simulink model "OttoCycle"  (R2018a)
settings: Solver=VariableStepAuto  StartTime=0.0  StopTime=0  RelTol=1e-3
settings Model: Creator=josefl  LastModifiedBy=josefl

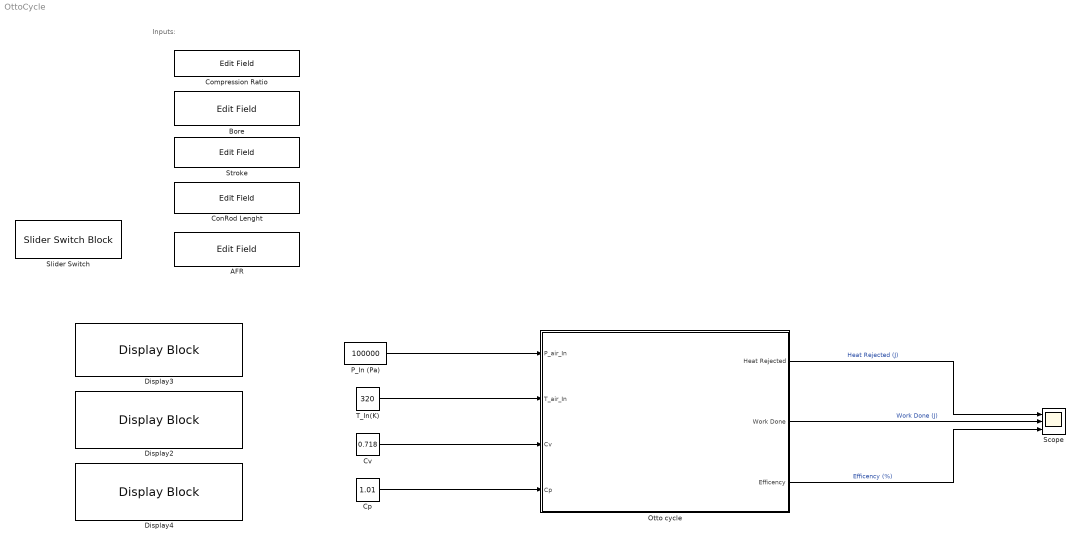
== system OttoCycle ==
  note: Inputs:
  AFR : EditField  WebBlockId=118  LabelPosition=Hide  Alignment=Center
  Bore : EditField  WebBlockId=61  LabelPosition=Hide  Alignment=Center
  "Compression Ratio " : EditField  WebBlockId=60  LabelPosition=Hide  Alignment=Center
  ConRod Lenght : EditField  WebBlockId=93  LabelPosition=Hide  Alignment=Center
  "Cp " : Constant  Value=1.01
  Cv : Constant  Value=0.718
  Display2 : DisplayBlock  WebBlockId=86
  Display3 : DisplayBlock  WebBlockId=87
  Display4 : DisplayBlock  WebBlockId=88
  "Otto cycle " : Subsystem
  "P_In (Pa) " : Constant  Value=100000
  Scope : Scope  NumInputPorts=3
  Slider Switch : SliderSwitchBlock  WebBlockId=121
      settings: Values={{'Off', 'On'}, [0.8 2]}
  "Stroke " : EditField  WebBlockId=62  LabelPosition=Hide  Alignment=Center
  "T_In(K) " : Constant  Value=320
  wires:
  Cv/1 -> "Otto cycle "/3(Cv)
  "Cp "/1 -> "Otto cycle "/4("Cp ")
  "Otto cycle "/1("Heat Rejected ") -> Scope/1  "Heat Rejected (J)"
  "Otto cycle "/2(Work Done) -> Scope/2  "Work Done (J)"
  "Otto cycle "/3(Efficency) -> Scope/3  "Efficency (%)"
  "T_In(K) "/1 -> "Otto cycle "/2("T_air_In ")
  "P_In (Pa) "/1 -> "Otto cycle "/1("P_air_In ")

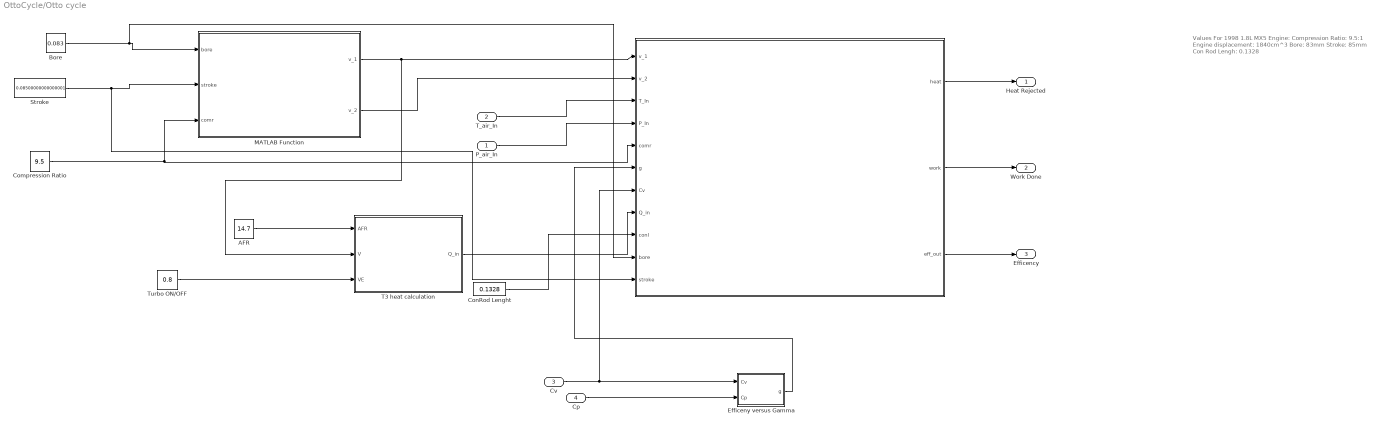
== system OttoCycle/Otto cycle  ==
  note: Values For 1998 1.8L MX5 Engine:
      | Compression Ratio: 9.5:1
      | Engine displacement: 1840cm^3
      | Bore: 83mm
      | Stroke: 85mm
      | Con Rod Lengh: 0.1328
  "P_air_In " : Inport
  "T_air_In " : Inport  Port=2
  Cv : Inport  Port=3
  "Cp " : Inport  Port=4
  " " : MATLAB Function  TreatAsAtomicUnit=on
  AFR : Constant  Value=14.7  VectorParams1D=off
  "Bore " : Constant  Value=0.083
  "Compression Ratio " : Constant  Value=9.5
  ConRod Lenght : Constant  Value=0.1328
  "Efficeny versus Gamma " : MATLAB Function  TreatAsAtomicUnit=on
  MATLAB Function : MATLAB Function  TreatAsAtomicUnit=on
  "Stroke " : Constant  Value=0.08500000000000001
  "T3 heat calculation " : MATLAB Function  TreatAsAtomicUnit=on
  "Turbo ON/OFF " : Constant  Value=0.8
  "Heat Rejected " : Outport
  Work Done : Outport  Port=2
  Efficency : Outport  Port=3
  wires:
  "Compression Ratio "/1 -> " "/5(comr), MATLAB Function/3(comr)
  "P_air_In "/1 -> " "/4(P_In)
  "T_air_In "/1 -> " "/3(T_In)
  Cv/1 -> " "/7(Cv), "Efficeny versus Gamma "/1(Cv)
  ConRod Lenght/1 -> " "/9(conl)
  "Cp "/1 -> "Efficeny versus Gamma "/2(Cp)
  " "/1(heat) -> "Heat Rejected "/1
  " "/2(work) -> Work Done/1
  " "/3(eff_out) -> Efficency/1
  "Efficeny versus Gamma "/1(g) -> " "/6(g)
  "T3 heat calculation "/1(Q_in) -> " "/8(Q_in)
  AFR/1 -> "T3 heat calculation "/1(AFR)
  "Turbo ON/OFF "/1 -> "T3 heat calculation "/3(VE)
  "Stroke "/1 -> " "/11(stroke), MATLAB Function/2(stroke)
  "Bore "/1 -> " "/10(bore), MATLAB Function/1(bore)
  MATLAB Function/1(v_1) -> "T3 heat calculation "/2(V), " "/1(v_1)
  MATLAB Function/2(v_2) -> " "/2(v_2)

== matlab function OttoCycle/Otto cycle /Efficeny versus Gamma  ==
  data: Cv input; g output; Cp input
function g = fcn(Cv,Cp)
r1 = 1:1:10;
g1 = 1.5;
g2 = 1.4;
g3 = 1.3;
g = Cp/Cv;
e1 = (1-(1./(r1)).^(g1-1))*100;
e2 = (1-(1./(r1)).^(g2-1))*100;
e3 = (1-(1./(r1)).^(g3-1))*100;
e = (1-(1./(r1)).^(g-1))*100;

figure(2);
hold on 
plot(r1,e1,'color','b');
plot(r1,e2,'color','g');
plot(r1,e3,'color','r');
plot(r1,e,'color','black');
xlabel('Compression Ratio');
ylabel('Efficiency');
title('Theoretical Otto Cycle Efficency');

== matlab function OttoCycle/Otto cycle /  ==
  data: v_1 input; v_2 input; T_In input; P_In input; comr input; g input; Cv input; Q_in input; conl input; heat output; work output; eff_out output; bore input; stroke input
function [heat,work,eff_out] = otto_cycle(v_1,v_2,T_In,P_In,comr,g,Cv,Q_in,conl,bore,stroke)

v_swept = (pi/4)*bore^2*stroke;
v_clearance = v_swept/(comr-1);
a = stroke/2;

%State 1
p1 = P_In;
v1 = v_1;
t1 = T_In;

%State 2 
v2 = v_2;
p2 = p1*((comr)^g);
t2 = t1*comr^(g-1);
c2 = p1*v1^g;

%Piston Kinematics
theta = linspace(0,180,100);
ka = conl./sind(theta);
B_ang = asind(a./ka);
C_ang = 180-(B_ang+theta);
x = ka.*sind(C_ang);
new_b = x-0.0903;

%Compression volume change
v_comp = ((pi/4)*bore^2.*new_b)+v_clearance;
p_comp = (c2./v_comp.^g);

%State 3 
v3 = v_2;
t3 = t2+(Q_in/Cv);
p3 = (p2*t3)/t2;
c3 = p3*v3^g;

%Expansion volume change
v_exp = v_comp;
p_exp = (c3./v_exp.^g);

%state 4 
v4 = v1;
p4 = p3/((comr)^g);
t4 = t3*(v3/v4)^(g-1);

%overview Calcs
heat = Cv*(t4-t1);
work = Q_in - heat;
eff = 1-(1/(comr)^(g-1));

%assigning output states 
eff_out = eff*100;

figure(1);
hold on
axis([0 0.0006 0 20000000])
plot(v1,p1,'*','color','r')
plot(v_comp,p_comp,'color','b')
plot(v2,p2,'*','color','r')
plot([v2 v3],[p2 p3],'color','b')
plot(v3,p3,'*','color','r')
plot(v_exp,p_exp,'color','b')
plot(v4,p4,'*','color','r')
plot([v4 v1],[p4 p1],'color','b')
xlabel('Volume in m^3')
ylabel('Pressure in Pa')
title('Theoretical Otto Cycle PV diagram');
grid on

== matlab function OttoCycle/Otto cycle /T3 heat calculation  ==
  data: Q_in output; AFR input; V input; VE input
function Q_in = heatadded(AFR,V,VE)

roh1 = 745;
roh2 = 1.2;
Va = AFR/roh2;
Vp = 1/roh1;
Vt = Va + Vp;
PercentageV = Vp/Vt;
V_used = V*VE;
MassFuel = (V_used*PercentageV)*roh1;
Q_in = 46400000*MassFuel;

== matlab function OttoCycle/Otto cycle /MATLAB Function ==
  data: bore input; v_1 output; stroke input; comr input; v_2 output
function [v_1,v_2] = volumeCalc(bore,stroke,comr)

v_swept = (pi/4)*bore^2*stroke;
v_2 = v_swept/(comr-1);
v_1 = v_swept + v_2;
